simulink model "SimulinkEulerAngleController"  (R2022a)
settings: Solver=VariableStepAuto  StartTime=0.0  StopTime=25  RelTol=1e-3
values from neighbouring files (symbols this model uses):
  D0 = 2 * sqrt(M0*(K0+K))    [EulerAngleController.m]
  dt = 0.01    [EulerAngleController.m]    (also in ex5mat.m)
  K0 = [1.5 0 0 ... (first row only)    [EulerAngleController.m]
  M0inv = inv(M0)    [EulerAngleController.m]
settings Model: Creator=Bruger  LastModifiedBy=Bruger

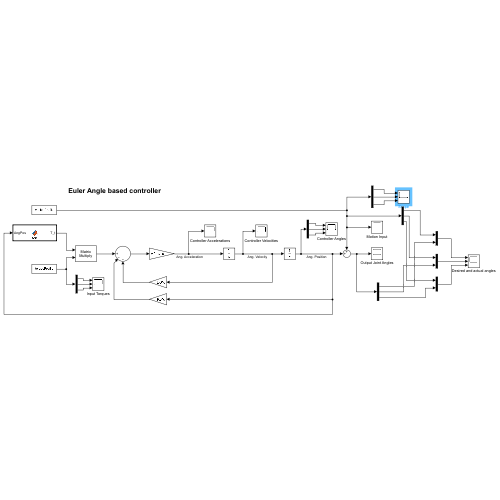
[thumbnail: Simulink's stored preview of the top-level diagram]
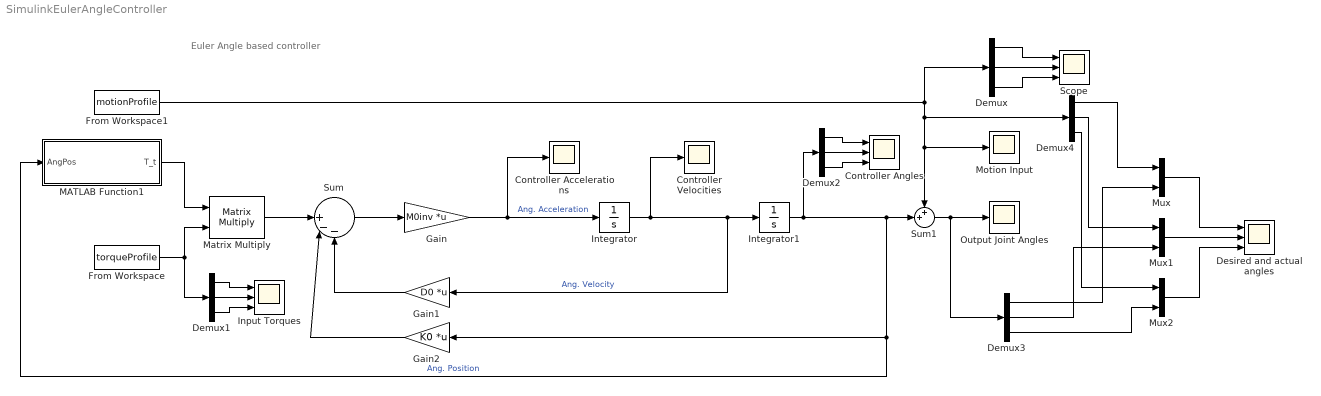
== system SimulinkEulerAngleController ==
  note: Euler Angle based controller
  Controller Accelerations : Scope
  Controller Angles : Scope  NumInputPorts=3
  Controller Velocities : Scope
  Demux{,1..4} (5 alike) : Demux  Outputs=3
  Desired and actual angles : Scope  NumInputPorts=3
  From Workspace : FromWorkspace  VariableName=torqueProfile
  From Workspace1 : FromWorkspace  VariableName=motionProfile  SampleTime=dt
  Gain : Gain  Gain=M0inv  Multiplication=Matrix(K*u)
  Gain1 : Gain  Gain=D0  Multiplication=Matrix(K*u)
  Gain2 : Gain  Gain=K0  Multiplication=Matrix(K*u)
  Input Torques : Scope  NumInputPorts=3
  Integrator : Integrator
  Integrator1 : Integrator
  MATLAB Function1 : MATLAB Function  TreatAsAtomicUnit=on
  Matrix Multiply : Product  Multiplication=Matrix(*)
  Motion Input : Scope
  Mux : Mux  Inputs=2
  Mux1 : Mux  Inputs=2
  Mux2 : Mux  Inputs=2
  Output Joint Angles : Scope
  Scope : Scope  NumInputPorts=3
  Sum : Sum  Inputs=||+--
  Sum1 : Sum  Inputs=++|
  wires:
  Gain/1 -> Controller Accelerations/1, Integrator/1  "Ang. Acceleration"
  Sum/1 -> Gain/1
  From Workspace1/1 -> Demux/1, Demux4/1, Sum1/1, Motion Input/1
  Integrator1/1 -> Demux2/1, Sum1/2, MATLAB Function1/1(AngPos), Gain2/1  "Ang. Position"
  Sum1/1 -> Demux3/1, Output Joint Angles/1
  Gain2/1 -> Sum/2
  Matrix Multiply/1 -> Sum/1
  Integrator/1 -> Integrator1/1, Gain1/1, Controller Velocities/1  "Ang. Velocity"
  Gain1/1 -> Sum/3
  MATLAB Function1/1(T_t) -> Matrix Multiply/1
  From Workspace/1 -> Demux1/1, Matrix Multiply/2
  Demux/2 -> Scope/2
  Demux/1 -> Scope/1
  Demux/3 -> Scope/3
  Demux1/1 -> Input Torques/1
  Demux1/2 -> Input Torques/2
  Demux1/3 -> Input Torques/3
  Demux2/1 -> Controller Angles/1
  Demux2/2 -> Controller Angles/2
  Demux2/3 -> Controller Angles/3
  Mux/1 -> Desired and actual angles/1
  Mux1/1 -> Desired and actual angles/2
  Mux2/1 -> Desired and actual angles/3
  Demux4/1 -> Mux/1
  Demux3/1 -> Mux/2
  Demux4/2 -> Mux1/1
  Demux3/2 -> Mux1/2
  Demux4/3 -> Mux2/1
  Demux3/3 -> Mux2/2

== matlab function SimulinkEulerAngleController/MATLAB Function1 ==
  data: AngPos input size=3; T_t output size=[3 3]
function T_t = fcn(AngPos)

% Takes the current angular position and calculates the angular position such that it can be integrated.

% The form of T only applies for ZYZ Euler angles. See lecture 5, slide 11
% for details.

T_t = [0 -sin(AngPos(1)) cos(AngPos(1))*sin(AngPos(2));
     0 cos(AngPos(1)) sin(AngPos(1))*sin(AngPos(2));
     1 0 cos(AngPos(2))]';
